simulink model "servoPotPrototype"  (R2023a)
settings: Solver=FixedStepAuto  StartTime=0.0  StopTime=inf  RelTol=1e-3  EnableMultiTasking=on
libraries: vexarmcortexlib x2
settings Model: ExtModeTrigDuration=25  Creator=bobsi  LastModifiedBy=bobsi
settings OptimizationCC: EnhancedBackFolding=on  PassReuseOutputArgsAs=Individual arguments  ZeroExternalMemoryAtStartup=off  ZeroInternalMemoryAtStartup=off  MaxStackSize=64  OptimizeBlockOrder=speed  DifferentSizesBufferReuse=on  OptimizationCustomize=off  EfficientTunableParamExpr=on
settings DebuggingCC: ParameterTunabilityLossMsg=error
settings HardwareCC: ProdBitPerPointer=32  ProdBitPerSizeT=32  ProdBitPerPtrDiffT=32  ProdLargestAtomicInteger=Long  ProdLargestAtomicFloat=Double  ProdWordSize=32  ProdHWDeviceType=ARM Compatible->ARM Cortex
settings SFSimCC: MATLABDynamicMemAlloc=off
settings RTWCC: Description=Embedded Coder  SystemTargetFile=ert.tlc  HardwareBoard=ARM Cortex-based VEX Microcontroller  TLCOptions="-aInlineSetEventsForThisBaseRateFcn=TLC_FALSE -aSuppressMultiTaskScheduler=TLC_FALSE  -aRateBasedStepFcn=0"  TemplateMakefile=ert_default_tmf  Toolchain=GNU Tools for VEX ARM Cortex
settings CodeAppCC: ForceParamTrailComments=on  IgnoreCustomStorageClasses=off  OperatorAnnotations=on  SimulinkDataObjDesc=on  SFDataObjDesc=on  InsertBlockDesc=on
settings ERTTargetCC: ExtModeTransport=1  ExtModeMexFile=ext_serial_win32_comm

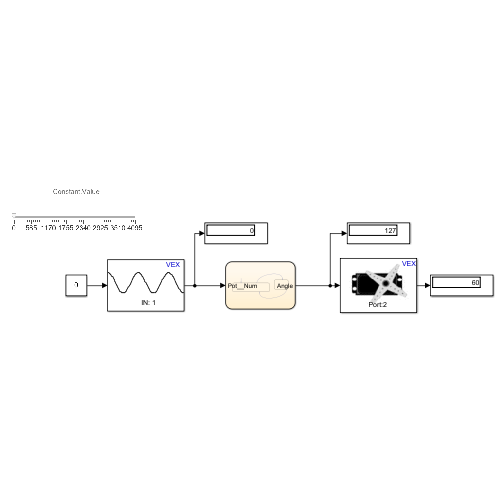
[thumbnail: Simulink's stored preview of the top-level diagram]
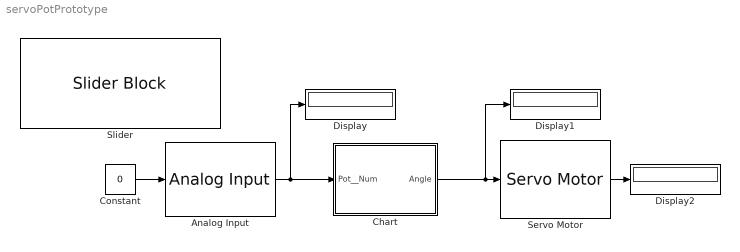
== system servoPotPrototype ==
  Analog Input : vexarmcortexlib/Sensors/Analog Input  inChan=1  SimulationIn=on  SampleTime=0.2
  Chart : Stateflow chart  TreatAsAtomicUnit=on
  Constant : Constant  Value=0
  Display : Display
  Display1 : Display
  Display2 : Display
  Servo Motor : vexarmcortexlib/Actuators/Servo Motor  motor=2  scaleFactor=60/127  SimulationOut=on
  Slider : SliderBlock  ScaleMax=4095
  wires:
  Constant/1 -> Analog Input/1
  Servo Motor/1 -> Display2/1
  Analog Input/1 -> Chart/1(Pot__Num), Display/1
  Chart/1(Angle) -> Display1/1, Servo Motor/1

== stateflow chart servoPotPrototype/Chart ==
  state Wait
    entry:
  state DIVIDE
    entry:
    Angle = 0-(Pot__Num-(4095/2))/(4095/(127*2));
  DIVIDE -> Wait : [after(0.1,sec)]
  (default) -> DIVIDE
  Wait -> DIVIDE : [after(0.1,sec)]
  data: Pot__Num input; Angle output
